simulink model "HybridSimulator"  (Simulink 7.5)
settings: Solver=ode45  StartTime=0.0  StopTime=T  MaxStep=MaxStep  RelTol=RelTol
values from neighbouring files (symbols this model uses):
  J = j(length(j))    [plotflows.m]    (also in run.m = 5)
  rule = 1    [run.m]
  T = t(length(t))    [plotflows.m]    (also in run.m = 1)
  x0 = [2;0.9;0]    [run.m]
undefined symbols (not defined in the file or in its folder): C, D, f, g, jumpPriority, O
libraries: simulink x2
CloseFcn:
  | rtwprivate ssgencode ModelCloseRequest HybridSimulator
settings Model: Creator=rsanfelice  LastModifiedBy=ricardo  ExtModeAutoUpdateStatusClock=off
settings SolverCC: ZeroCrossControl=DisableAll
settings DataIOCC: LimitDataPoints=off  SaveOutput=off  SignalLogging=off  DSMLogging=off  SaveTime=off
settings OptimizationCC: EnhancedBackFolding=on  InitFltsAndDblsToZero=on  SimCompilerOptimization=On
settings DebuggingCC: AlgebraicLoopMsg=none  SaveWithParameterizedLinksMsg=none  SignalResolutionControl=TryResolveAllWithWarning  SolverPrmCheckMsg=none  MultiTaskDSMMsg=warning  MultiTaskCondExecSysMsg=none  StrictBusMsg=None
settings HardwareCC: TargetIntDivRoundTo=Zero  TargetEndianess=LittleEndian  TargetHWDeviceType=MATLAB Host  ProdEqTarget=off
settings RTWCC: IncludeERTFirstTime=on
settings GRTTargetCC: TargetFcnLib=ansi_tfl_tmw.mat

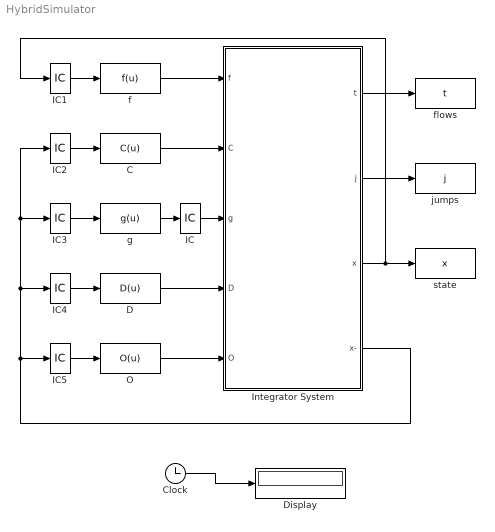
== system HybridSimulator ==
  C : MATLABFcn  MATLABFcn=C(u)
  Clock : Clock
      settings: Decimation=10
  D : MATLABFcn  MATLABFcn=D(u)
  Display : Display
  IC{,1..5} (6 alike) : InitialCondition  Value=x0
  Integrator System : Subsystem
  O : MATLABFcn  MATLABFcn=O(u)
  f : MATLABFcn  MATLABFcn=f(u)
  flows : ToWorkspace  VariableName=t  SampleTime=-1  SaveFormat=Array
  g : MATLABFcn  MATLABFcn=g(u)
  jumps : ToWorkspace  VariableName=j  SampleTime=-1  SaveFormat=Array
  state : ToWorkspace  VariableName=x  SampleTime=-1  SaveFormat=Array
  wires:
  f/1 -> Integrator System/1(f)
  Integrator System/4(x-) -> IC2/1, IC3/1, IC4/1, IC5/1
  Integrator System/3(x) -> state/1, IC1/1
  C/1 -> Integrator System/2(C)
  Integrator System/1(t) -> flows/1
  Integrator System/2(j) -> jumps/1
  O/1 -> Integrator System/5(O)
  IC1/1 -> f/1
  IC5/1 -> O/1
  IC4/1 -> D/1
  IC3/1 -> g/1
  IC2/1 -> C/1
  D/1 -> Integrator System/4(D)
  g/1 -> IC/1
  IC/1 -> Integrator System/3(g)
  Clock/1 -> Display/1

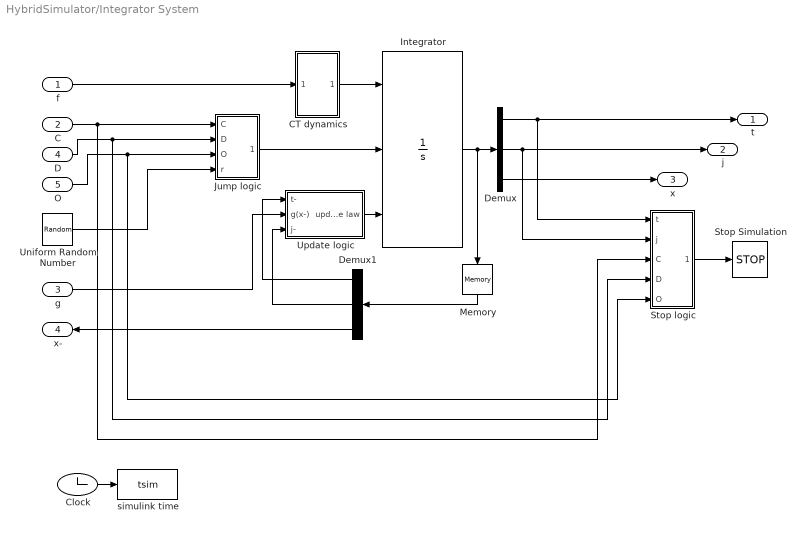
== system HybridSimulator/Integrator System ==
  f : Inport
  C : Inport  Port=2
  g : Inport  Port=3
  D : Inport  Port=4
  O : Inport  Port=5
  CT dynamics : Subsystem
  Clock : Clock
      settings: Decimation=10
  Demux : Demux  Outputs=[1 1 -1]
  Demux1 : Demux  Outputs=[1 1 -1]
  Integrator : Integrator  ExternalReset=level hold  InitialConditionSource=external  ZeroCross=off
  Jump logic : Subsystem
  Memory : Memory
  Stop Simulation : Stop
  Stop logic : Subsystem
  Uniform Random Number : UniformRandomNumber  Minimum=0  Seed=abs(floor(100*rand))  SampleTime=0
  Update logic : Subsystem
  simulink time : ToWorkspace  VariableName=tsim  SampleTime=-1  SaveFormat=Array
  t : Outport
  j : Outport  Port=2
  x : Outport  Port=3
  x- : Outport  Port=4
  wires:
  Demux/2 -> j/1, Stop logic/2(j)
  Demux/1 -> t/1, Stop logic/1(t)
  Demux1/2 -> Update logic/3(j-)
  Demux1/1 -> Update logic/1(t-)
  Update logic/1(update law) -> Integrator/3
  CT dynamics/1(dot) -> Integrator/1
  Stop logic/1(stop) -> Stop Simulation/1
  Integrator/1 -> Demux/1, Memory/1
  C/1 -> Jump logic/1(C), Stop logic/3(C)
  D/1 -> Jump logic/2(D), Stop logic/4(D)
  O/1 -> Jump logic/3(O), Stop logic/5(O)
  f/1 -> CT dynamics/1(f(x))
  Demux1/3 -> x-/1
  Clock/1 -> simulink time/1
  g/1 -> Update logic/2(g(x-))
  Jump logic/1(jump) -> Integrator/2
  Uniform Random Number/1 -> Jump logic/4(r)
  Demux/3 -> x/1
  Memory/1 -> Demux1/1

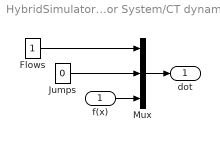
== system HybridSimulator/Integrator System/CT dynamics ==
  f(x) : Inport
  Flows : Constant
  Jumps : Constant  Value=0
  Mux : Mux  Inputs=[1 1 -1]
  dot : Outport
  wires:
  Jumps/1 -> Mux/2
  Flows/1 -> Mux/1
  Mux/1 -> dot/1
  f(x)/1 -> Mux/3

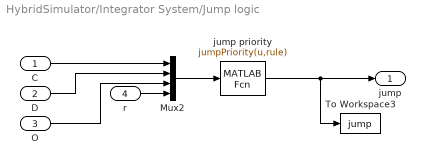
== system HybridSimulator/Integrator System/Jump logic ==
  C : Inport
  D : Inport  Port=2
  O : Inport  Port=3
  r : Inport  Port=4
  Mux2 : Mux
  To Workspace3 : ToWorkspace  VariableName=jump  SampleTime=-1  SaveFormat=Array
  jump priority : MATLABFcn  MATLABFcn=jumpPriority(u,rule)
  jump : Outport
  wires:
  Mux2/1 -> jump priority/1
  jump priority/1 -> jump/1, To Workspace3/1
  C/1 -> Mux2/1
  r/1 -> Mux2/4
  D/1 -> Mux2/2
  O/1 -> Mux2/3

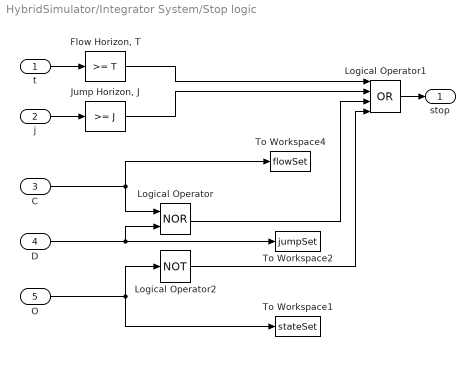
== system HybridSimulator/Integrator System/Stop logic ==
  t : Inport
  j : Inport  Port=2
  C : Inport  Port=3
  D : Inport  Port=4
  O : Inport  Port=5
  "Flow Horizon, T" : simulink/Logic and Bit Operations/Compare To Constant  SystemSampleTime=-1  relop=>=  const=T  LogicOutDataTypeMode=uint8  ZeroCross=off
  "Jump Horizon, J" : simulink/Logic and Bit Operations/Compare To Constant  SystemSampleTime=-1  relop=>=  const=J  LogicOutDataTypeMode=uint8  ZeroCross=off
  Logical Operator : Logic  Operator=NOR  AllPortsSameDT=off  OutDataTypeMode=boolean  OutDataTypeStr=boolean
  Logical Operator1 : Logic  Operator=OR  Inputs=4  AllPortsSameDT=off  OutDataTypeMode=boolean  OutDataTypeStr=boolean
  Logical Operator2 : Logic  Operator=NOT  AllPortsSameDT=off  OutDataTypeMode=boolean  OutDataTypeStr=boolean
  To Workspace1 : ToWorkspace  VariableName=stateSet  SampleTime=-1  SaveFormat=Array
  To Workspace2 : ToWorkspace  VariableName=jumpSet  SampleTime=-1  SaveFormat=Array
  To Workspace4 : ToWorkspace  VariableName=flowSet  SampleTime=-1  SaveFormat=Array
  stop : Outport
  wires:
  "Flow Horizon, T"/1 -> Logical Operator1/1
  "Jump Horizon, J"/1 -> Logical Operator1/2
  Logical Operator/1 -> Logical Operator1/3
  Logical Operator2/1 -> Logical Operator1/4
  D/1 -> Logical Operator/2, To Workspace2/1
  O/1 -> Logical Operator2/1, To Workspace1/1
  t/1 -> "Flow Horizon, T"/1
  j/1 -> "Jump Horizon, J"/1
  C/1 -> Logical Operator/1, To Workspace4/1
  Logical Operator1/1 -> stop/1

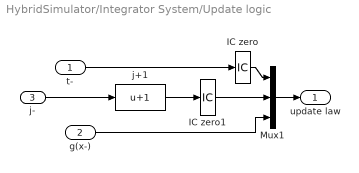
== system HybridSimulator/Integrator System/Update logic ==
  t- : Inport
  g(x-) : Inport  Port=2
  j- : Inport  Port=3
  IC zero : InitialCondition  Value=0
  IC zero1 : InitialCondition  Value=0
  Mux1 : Mux  Inputs=[1 1 -1]
  j+1 : MATLABFcn  MATLABFcn=u+1
  update law : Outport
  wires:
  IC zero1/1 -> Mux1/2
  j+1/1 -> IC zero1/1
  IC zero/1 -> Mux1/1
  t-/1 -> IC zero/1
  Mux1/1 -> update law/1
  j-/1 -> j+1/1
  g(x-)/1 -> Mux1/3
